simulink model "Simulation_6DOF"  (R2024a)
settings: Solver=ode4  StartTime=initial_time  StopTime=final_time  FixedStep=timestep  RelTol=1e-3
values from neighbouring files (symbols this model uses):
  aEarth = 0    [CodeTesting_6DOF.m]    (also in Constants_6DOF.m = 6378137; Constants_6DOFTesting.m = 6378137)
  alphaArray = [-30, -25, -20, -15, -10, -5, 0, 5, 10, 15, 20, 25, 30]    [CodeTesting_6DOF.m]    (also in Constants_6DOF.m; Constants_6DOFTesting.m)
  altitudeArray = [0, 1000, 2000, 3000, 4000, 5000, 6000, 7000, 8000, 9000, 10000, 15000, 20000,      25000, 30000, 35000, 40000, 45000, 50000, 55000, 60000]    [CodeTesting_6DOF.m]    (also in Constants_6DOF.m; Constants_6DOFTesting.m)
  AoA0Wind = 0    [CodeTesting_6DOF.m]    (also in Constants_6DOF.m = deg2rad(AoA0Wind); Constants_6DOFTesting.m = deg2rad(AoA0Wind))
  bEarth = 0    [CodeTesting_6DOF.m]    (also in Constants_6DOF.m = 6356752.3; Constants_6DOFTesting.m = 6356752.3)
  cD_3DArray = zeros(numAoAs, numMachs, numAltitudes)    [CodeTesting_6DOF.m]    (also in Constants_6DOF.m; Constants_6DOFTesting.m)
  cL_3DArray = zeros(numAoAs, numMachs, numAltitudes)    [CodeTesting_6DOF.m]    (also in Constants_6DOF.m; Constants_6DOFTesting.m)
  densityList = rhoList    [CodeTesting_6DOF.m]    (also in Constants_6DOF.m = usAtmosphere.x_; Constants_6DOFTesting.m = usAtmosphere.x_)
  heightsList = usAtmosphere.Z    [CodeTesting_6DOF.m]    (also in Constants_6DOF.m; Constants_6DOFTesting.m)
  Ixx = 10    [CodeTesting_6DOF.m]    (also in Constants_6DOF.m; Constants_6DOFTesting.m = 4.88094462)
  Ixz = 10    [CodeTesting_6DOF.m]    (also in Constants_6DOF.m = 1; Constants_6DOFTesting.m = 4.88094462)
  Iyy = 10    [CodeTesting_6DOF.m]    (also in Constants_6DOF.m; Constants_6DOFTesting.m = 4.88094462)
  Izz = 10    [CodeTesting_6DOF.m]    (also in Constants_6DOF.m; Constants_6DOFTesting.m = 4.88094462)
  latitude0 = pi/4    (= 0.785398163397)    [CodeTesting_6DOF.m]    (also in Constants_6DOF.m = deg2rad(latitude0); Constants_6DOFTesting.m = deg2rad(latitude0))
  longitude0 = pi/4    (= 0.785398163397)    [CodeTesting_6DOF.m]    (also in Constants_6DOF.m = deg2rad(longitude0); Constants_6DOFTesting.m = deg2rad(longitude0))
  m0 = 10    [CodeTesting_6DOF.m]    (also in Constants_6DOF.m = 50; Constants_6DOFTesting.m = 14.5939029)
  machArray = [0.5, 1.0, 1.5, 2.0, 2.5, 3.0, 3.5, 4.0, 4.5, 5.0, 5.5, 6.0, 6.5, 7.0, 7.5, 8.0,      8.5, 9.0, 9.5, 10.0]    [CodeTesting_6DOF.m]    (also in Constants_6DOF.m; Constants_6DOFTesting.m)
  omegaEarth = omega_earth    (= 7.2921159e-05)    [CodeTesting_6DOF.m]    (also in Constants_6DOF.m; Constants_6DOFTesting.m)
  p0Wind = 0    [CodeTesting_6DOF.m]    (also in Constants_6DOF.m = deg2rad(p0Wind))
  q0Wind = 0    [CodeTesting_6DOF.m]    (also in Constants_6DOF.m = deg2rad(q0Wind))
  r0Wind = 0    [CodeTesting_6DOF.m]    (also in Constants_6DOF.m = deg2rad(r0Wind))
  rEarth = r_earth    (= 6371008.8)    [CodeTesting_6DOF.m]    (also in Constants_6DOF.m; Constants_6DOFTesting.m)
  rollAngle0Wind = 0    [CodeTesting_6DOF.m]    (also in Constants_6DOF.m = deg2rad(rollAngle0Wind); Constants_6DOFTesting.m = deg2rad(rollAngle0Wind))
  sideslipAngle0Wind = 0    [CodeTesting_6DOF.m]    (also in Constants_6DOF.m = deg2rad(sideslipAngle0Wind); Constants_6DOFTesting.m = deg2rad(sideslipAngle0Wind))
  temperatureList = usAtmosphere.T    [CodeTesting_6DOF.m]    (also in Constants_6DOF.m; Constants_6DOFTesting.m)
  u0Wind = 5    [CodeTesting_6DOF.m]    (also in Constants_6DOF.m)
  v0Wind = 5    [CodeTesting_6DOF.m]    (also in Constants_6DOF.m = 0)
  w0Wind = 0    [CodeTesting_6DOF.m]    (also in Constants_6DOF.m)
  wingArea = 0    [CodeTesting_6DOF.m]    (also in Constants_6DOF.m = 50; Constants_6DOFTesting.m = 0.09290304)
  x0Wind = 5    [CodeTesting_6DOF.m]    (also in Constants_6DOF.m = 0)
  y0Wind = 5    [CodeTesting_6DOF.m]    (also in Constants_6DOF.m = 0)
  z0Wind = 5    [CodeTesting_6DOF.m]    (also in Constants_6DOF.m = 0)
settings Model: Creator=641893  LastModifiedBy=641893

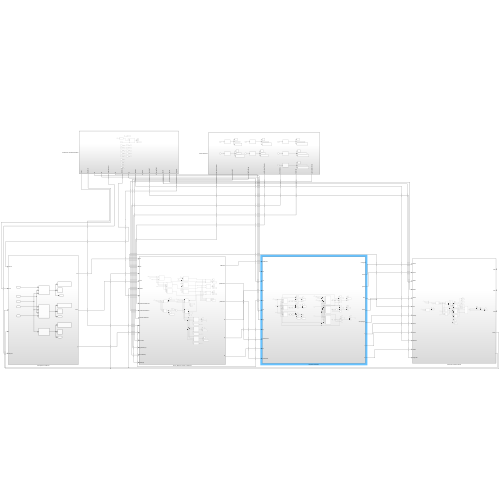
[thumbnail: Simulink's stored preview of the top-level diagram]
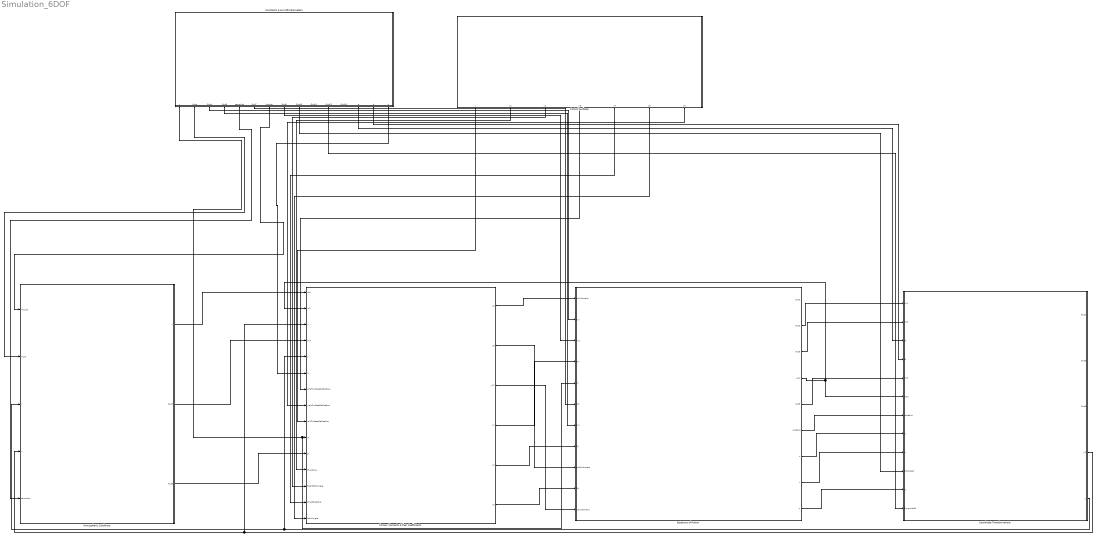
== system Simulation_6DOF ==
  Atmospheric Conditions : Subsystem
  Constants & Aircraft Parameters : Subsystem
  Control Surfaces : Subsystem
  Coordinate Transformations : Subsystem
  Equations of Motion : Subsystem
  "Forces, Moments & their Coefficients" : Subsystem
  wires:
  Atmospheric Conditions/1(y) -> "Forces, Moments & their Coefficients"/1(rho)
  Atmospheric Conditions/2(Out2) -> "Forces, Moments & their Coefficients"/4(In4)
  Atmospheric Conditions/3(Out3) -> "Forces, Moments & their Coefficients"/11(g)
  Equations of Motion/4(AoA) -> Coordinate Transformations/6(AoA), "Forces, Moments & their Coefficients"/2(In2)
  Constants & Aircraft Parameters/7(rhoList) -> Atmospheric Conditions/1(rhoList)
  Constants & Aircraft Parameters/2(hList) -> Atmospheric Conditions/2(hList)
  Constants & Aircraft Parameters/5(tempList) -> Atmospheric Conditions/5(tempList)
  Coordinate Transformations/4(y4) -> "Forces, Moments & their Coefficients"/3(v), Atmospheric Conditions/4(v)
  Coordinate Transformations/5(y) -> "Forces, Moments & their Coefficients"/5(y), Atmospheric Conditions/3(r)
  Constants & Aircraft Parameters/15(A) -> "Forces, Moments & their Coefficients"/6(A)
  Constants & Aircraft Parameters/1(y) -> Equations of Motion/5(m), "Forces, Moments & their Coefficients"/10(m)
  Control Surfaces/1(y) -> "Forces, Moments & their Coefficients"/9(rollSurfaceDeflection)
  Control Surfaces/4(y3) -> "Forces, Moments & their Coefficients"/7(pitchSurfaceDeflection)
  Control Surfaces/7(y6) -> "Forces, Moments & their Coefficients"/8(yawSurfaceDeflection)
  Control Surfaces/2(y1) -> "Forces, Moments & their Coefficients"/12(thrustAoA)
  Control Surfaces/3(y2) -> "Forces, Moments & their Coefficients"/13(flightPathAngle)
  Control Surfaces/5(y4) -> "Forces, Moments & their Coefficients"/14(thrustSideslip)
  Control Surfaces/6(y5) -> "Forces, Moments & their Coefficients"/15(bankAngle)
  "Forces, Moments & their Coefficients"/1(y5) -> Equations of Motion/1(rollMoment)
  "Forces, Moments & their Coefficients"/2(y8) -> Equations of Motion/9(pitchMoment)
  "Forces, Moments & their Coefficients"/3(y11) -> Equations of Motion/11(yawMoment)
  "Forces, Moments & their Coefficients"/6(y3) -> Equations of Motion/10(Fz)
  "Forces, Moments & their Coefficients"/5(y2) -> Equations of Motion/8(Fy)
  "Forces, Moments & their Coefficients"/4(y1) -> Equations of Motion/4(Fx)
  Constants & Aircraft Parameters/3(Out4) -> Equations of Motion/2(Ixx)
  Constants & Aircraft Parameters/4(Out5) -> Equations of Motion/7(Iyy)
  Constants & Aircraft Parameters/6(Out7) -> Equations of Motion/6(Izz)
  Constants & Aircraft Parameters/8(Out9) -> Equations of Motion/3(Ixz)
  Equations of Motion/2(Out2) -> Coordinate Transformations/1(In1)
  Equations of Motion/3(Out3) -> Coordinate Transformations/2(In3)
  Equations of Motion/5(Out5) -> Coordinate Transformations/5(In8)
  Equations of Motion/6(sideslip) -> Coordinate Transformations/7(sideslip)
  Equations of Motion/7(u) -> Coordinate Transformations/8(u)
  Equations of Motion/8(v) -> Coordinate Transformations/9(v)
  Equations of Motion/9(w) -> Coordinate Transformations/11(w)
  Constants & Aircraft Parameters/9(Out10) -> Coordinate Transformations/10(latitude0)
  Constants & Aircraft Parameters/13(a) -> Coordinate Transformations/3(a)
  Constants & Aircraft Parameters/14(b) -> Coordinate Transformations/4(b)
  Constants & Aircraft Parameters/11(Out12) -> Coordinate Transformations/12(longitude0)

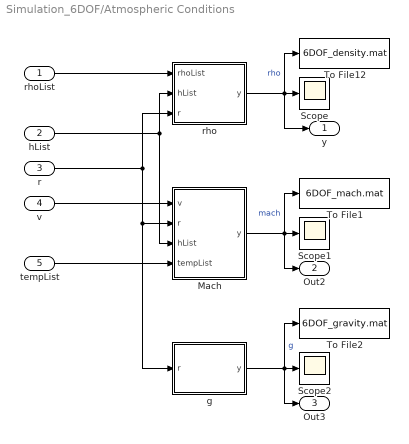
== system Simulation_6DOF/Atmospheric Conditions ==
  rhoList : Inport
  hList : Inport  Port=2
  r : Inport  Port=3
  v : Inport  Port=4
  tempList : Inport  Port=5
  Mach : MATLAB Function  TreatAsAtomicUnit=on
  Scope : Scope
  Scope1 : Scope
  Scope2 : Scope
  To File1 : ToFile  Filename=6DOF_mach.mat
  To File12 : ToFile  Filename=6DOF_density.mat
  To File2 : ToFile  Filename=6DOF_gravity.mat
  g : MATLAB Function  TreatAsAtomicUnit=on
  rho : MATLAB Function  TreatAsAtomicUnit=on
  y : Outport
  Out2 : Outport  Port=2
  Out3 : Outport  Port=3
  wires:
  rho/1(y) -> Scope/1, To File12/1, y/1  "rho"
  Mach/1(y) -> Scope1/1, To File1/1, Out2/1  "mach"
  g/1(y) -> To File2/1, Scope2/1, Out3/1  "g"
  hList/1 -> rho/2(hList), Mach/3(hList)
  v/1 -> Mach/1(v)
  tempList/1 -> Mach/4(tempList)
  r/1 -> rho/3(r), g/1(r), Mach/2(r)
  rhoList/1 -> rho/1(rhoList)

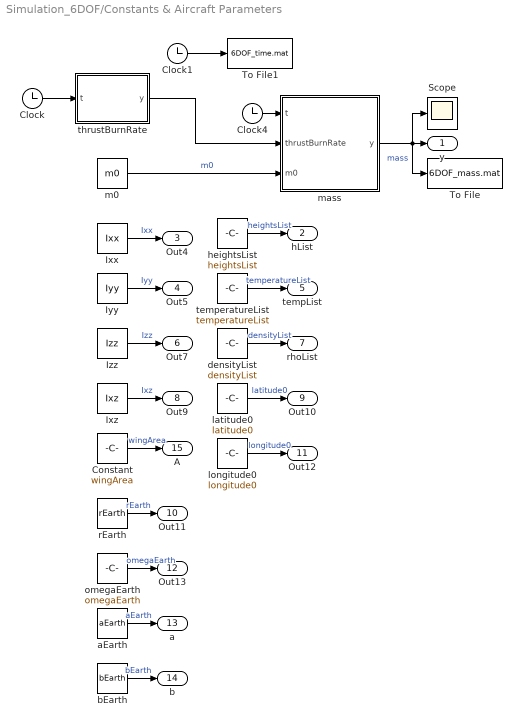
== system Simulation_6DOF/Constants & Aircraft Parameters ==
  Clock : Clock
  Clock1 : Clock
  Clock4 : Clock
  Constant : Constant  Value=wingArea
  Ixx : Constant  Value=Ixx
  Ixz : Constant  Value=Ixz
  Iyy : Constant  Value=Iyy
  Izz : Constant  Value=Izz
  Scope : Scope
  To File : ToFile  Filename=6DOF_mass.mat
  To File1 : ToFile  Filename=6DOF_time.mat
  aEarth : Constant  Value=aEarth
  bEarth : Constant  Value=bEarth
  densityList : Constant  Value=densityList
  heightsList : Constant  Value=heightsList
  latitude0 : Constant  Value=latitude0
  longitude0 : Constant  Value=longitude0
  m0 : Constant  Value=m0
  mass : MATLAB Function  TreatAsAtomicUnit=on
  omegaEarth : Constant  Value=omegaEarth
  rEarth : Constant  Value=rEarth
  temperatureList : Constant  Value=temperatureList
  thrustBurnRate : MATLAB Function  TreatAsAtomicUnit=on
  y : Outport
  hList : Outport  Port=2
  Out4 : Outport  Port=3
  Out5 : Outport  Port=4
  tempList : Outport  Port=5
  Out7 : Outport  Port=6
  rhoList : Outport  Port=7
  Out9 : Outport  Port=8
  Out10 : Outport  Port=9
  Out11 : Outport  Port=10
  Out12 : Outport  Port=11
  Out13 : Outport  Port=12
  a : Outport  Port=13
  b : Outport  Port=14
  A : Outport  Port=15
  wires:
  m0/1 -> mass/3(m0)  "m0"
  Clock4/1 -> mass/1(t)
  heightsList/1 -> hList/1  "heightsList"
  Clock/1 -> thrustBurnRate/1(t)
  omegaEarth/1 -> Out13/1  "omegaEarth"
  thrustBurnRate/1(y) -> mass/2(thrustBurnRate)
  rEarth/1 -> Out11/1  "rEarth"
  latitude0/1 -> Out10/1  "latitude0"
  mass/1(y) -> To File/1, Scope/1, y/1  "mass"
  aEarth/1 -> a/1  "aEarth"
  densityList/1 -> rhoList/1  "densityList"
  longitude0/1 -> Out12/1  "longitude0"
  bEarth/1 -> b/1  "bEarth"
  Izz/1 -> Out7/1  "Izz"
  Ixz/1 -> Out9/1  "Ixz"
  Ixx/1 -> Out4/1  "Ixx"
  temperatureList/1 -> tempList/1  "temperatureList"
  Iyy/1 -> Out5/1  "Iyy"
  Constant/1 -> A/1  "wingArea"
  Clock1/1 -> To File1/1

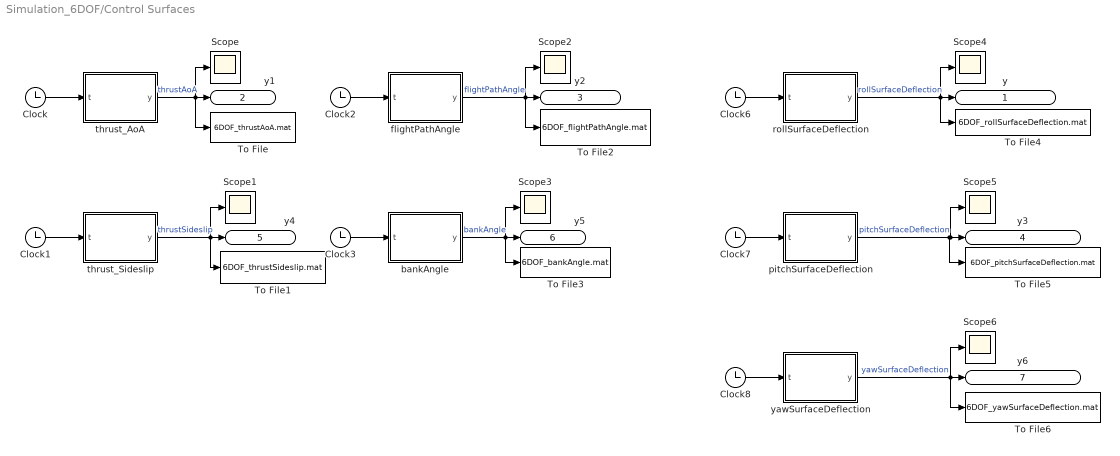
== system Simulation_6DOF/Control Surfaces ==
  Clock{,1..3,6..8} (7 alike) : Clock
  Scope{,1..6} (7 alike) : Scope
  To File : ToFile  Filename=6DOF_thrustAoA.mat
  To File1 : ToFile  Filename=6DOF_thrustSideslip.mat
  To File2 : ToFile  Filename=6DOF_flightPathAngle.mat
  To File3 : ToFile  Filename=6DOF_bankAngle.mat
  To File4 : ToFile  Filename=6DOF_rollSurfaceDeflection.mat
  To File5 : ToFile  Filename=6DOF_pitchSurfaceDeflection.mat
  To File6 : ToFile  Filename=6DOF_yawSurfaceDeflection.mat
  bankAngle : MATLAB Function  TreatAsAtomicUnit=on
  flightPathAngle : MATLAB Function  TreatAsAtomicUnit=on
  pitchSurfaceDeflection : MATLAB Function  TreatAsAtomicUnit=on
  rollSurfaceDeflection : MATLAB Function  TreatAsAtomicUnit=on
  thrust_AoA : MATLAB Function  TreatAsAtomicUnit=on
  thrust_Sideslip : MATLAB Function  TreatAsAtomicUnit=on
  yawSurfaceDeflection : MATLAB Function  TreatAsAtomicUnit=on
  y : Outport
  y1 : Outport  Port=2
  y2 : Outport  Port=3
  y3 : Outport  Port=4
  y4 : Outport  Port=5
  y5 : Outport  Port=6
  y6 : Outport  Port=7
  wires:
  Clock8/1 -> yawSurfaceDeflection/1(t)
  rollSurfaceDeflection/1(y) -> Scope4/1, y/1, To File4/1  "rollSurfaceDeflection"
  Clock1/1 -> thrust_Sideslip/1(t)
  bankAngle/1(y) -> Scope3/1, y5/1, To File3/1  "bankAngle"
  Clock6/1 -> rollSurfaceDeflection/1(t)
  Clock7/1 -> pitchSurfaceDeflection/1(t)
  pitchSurfaceDeflection/1(y) -> To File5/1, Scope5/1, y3/1  "pitchSurfaceDeflection"
  Clock2/1 -> flightPathAngle/1(t)
  thrust_AoA/1(y) -> Scope/1, y1/1, To File/1  "thrustAoA"
  Clock/1 -> thrust_AoA/1(t)
  Clock3/1 -> bankAngle/1(t)
  thrust_Sideslip/1(y) -> Scope1/1, y4/1, To File1/1  "thrustSideslip"
  flightPathAngle/1(y) -> Scope2/1, y2/1, To File2/1  "flightPathAngle"
  yawSurfaceDeflection/1(y) -> Scope6/1, y6/1, To File6/1  "yawSurfaceDeflection"

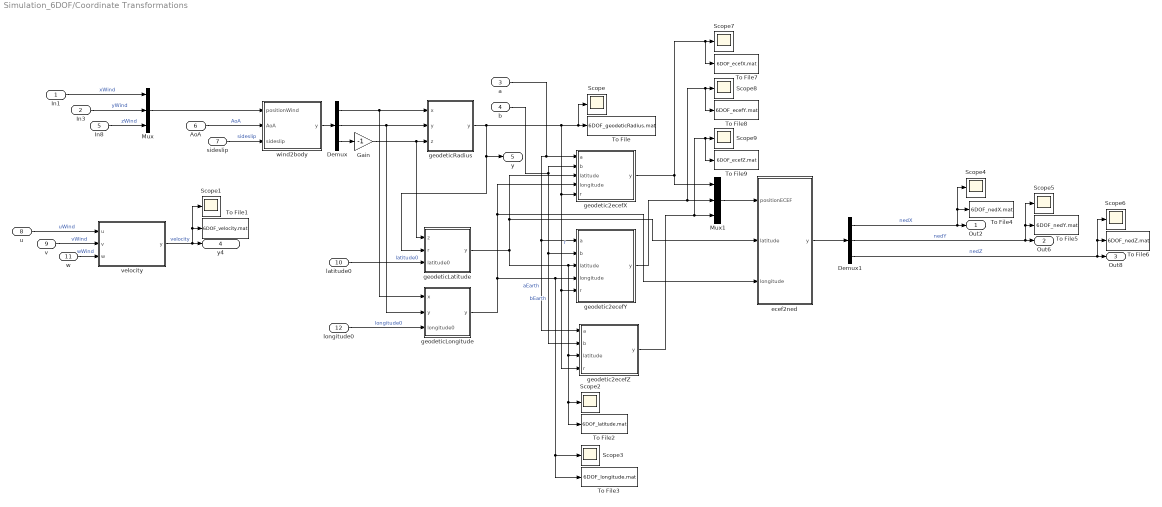
== system Simulation_6DOF/Coordinate Transformations ==
  In1 : Inport
  In3 : Inport  Port=2
  a : Inport  Port=3
  b : Inport  Port=4
  In8 : Inport  Port=5
  AoA : Inport  Port=6
  sideslip : Inport  Port=7
  u : Inport  Port=8
  v : Inport  Port=9
  latitude0 : Inport  Port=10
  w : Inport  Port=11
  longitude0 : Inport  Port=12
  Demux : Demux  Outputs=3
  Demux1 : Demux  Outputs=3
  Gain : Gain  Gain=-1
  Mux : Mux  Inputs=3
  Mux1 : Mux  Inputs=3
  Scope{,1..9} (10 alike) : Scope
  To File : ToFile  Filename=6DOF_geodeticRadius.mat
  To File1 : ToFile  Filename=6DOF_velocity.mat
  To File2 : ToFile  Filename=6DOF_latitude.mat
  To File3 : ToFile  Filename=6DOF_longitude.mat
  To File4 : ToFile  Filename=6DOF_nedX.mat
  To File5 : ToFile  Filename=6DOF_nedY.mat
  To File6 : ToFile  Filename=6DOF_nedZ.mat
  To File7 : ToFile  Filename=6DOF_ecefX.mat
  To File8 : ToFile  Filename=6DOF_ecefY.mat
  To File9 : ToFile  Filename=6DOF_ecefZ.mat
  ecef2ned : MATLAB Function  TreatAsAtomicUnit=on
  geodetic2ecefX : MATLAB Function  TreatAsAtomicUnit=on
  geodetic2ecefY : MATLAB Function  TreatAsAtomicUnit=on
  geodetic2ecefZ : MATLAB Function  TreatAsAtomicUnit=on
  geodeticLatitude : MATLAB Function  TreatAsAtomicUnit=on
  geodeticLongitude : MATLAB Function  TreatAsAtomicUnit=on
  geodeticRadius : MATLAB Function  TreatAsAtomicUnit=on
  velocity : MATLAB Function  TreatAsAtomicUnit=on
  wind2body : MATLAB Function  TreatAsAtomicUnit=on
  Out2 : Outport
  Out6 : Outport  Port=2
  Out8 : Outport  Port=3
  y4 : Outport  Port=4
  y : Outport  Port=5
  wires:
  Mux/1 -> wind2body/1(positionWind)
  geodeticRadius/1(y) -> y/1, geodeticLatitude/2(r), Scope/1, To File/1, geodetic2ecefX/5(r), geodetic2ecefY/5(r), geodetic2ecefZ/4(r)  "r"
  ecef2ned/1(y) -> Demux1/1
  v/1 -> velocity/2(v)  "vWind"
  u/1 -> velocity/1(u)  "uWind"
  sideslip/1 -> wind2body/3(sideslip)  "sideslip"
  Demux1/1 -> Scope4/1, To File4/1, Out2/1  "nedX"
  wind2body/1(y) -> Demux/1
  geodeticLongitude/1(y) -> geodetic2ecefY/4(longitude), Scope3/1, To File3/1, geodetic2ecefX/4(longitude), ecef2ned/3(longitude)
  b/1 -> geodetic2ecefX/2(b), geodetic2ecefY/2(b), geodetic2ecefZ/2(b)  "bEarth"
  longitude0/1 -> geodeticLongitude/3(longitude0)  "longitude0"
  Demux1/3 -> Scope6/1, To File6/1, Out8/1  "nedZ"
  Demux/3 -> Gain/1
  Demux1/2 -> Scope5/1, To File5/1, Out6/1  "nedY"
  latitude0/1 -> geodeticLatitude/3(latitude0)  "latitude0"
  a/1 -> geodetic2ecefX/1(a), geodetic2ecefZ/1(a), geodetic2ecefY/1(a)  "aEarth"
  w/1 -> velocity/3(w)  "wWind"
  AoA/1 -> wind2body/2(AoA)  "AoA"
  geodeticLatitude/1(y) -> geodetic2ecefZ/3(latitude), To File2/1, Scope2/1, geodetic2ecefY/3(latitude), geodetic2ecefX/3(latitude), ecef2ned/2(latitude)
  Demux/1 -> geodeticLongitude/1(x), geodeticRadius/1(x)
  Demux/2 -> geodeticRadius/2("y "), geodeticLongitude/2("y ")
  In8/1 -> Mux/3  "zWind"
  In1/1 -> Mux/1  "xWind"
  velocity/1(y) -> Scope1/1, To File1/1, y4/1  "velocity"
  In3/1 -> Mux/2  "yWind"
  Mux1/1 -> ecef2ned/1(positionECEF)
  geodetic2ecefX/1(y) -> To File7/1, Scope7/1, Mux1/1
  geodetic2ecefY/1(y) -> Mux1/2, To File8/1, Scope8/1
  geodetic2ecefZ/1(y) -> Mux1/3, To File9/1, Scope9/1
  Gain/1 -> geodeticLatitude/1(z), geodeticRadius/3(z)

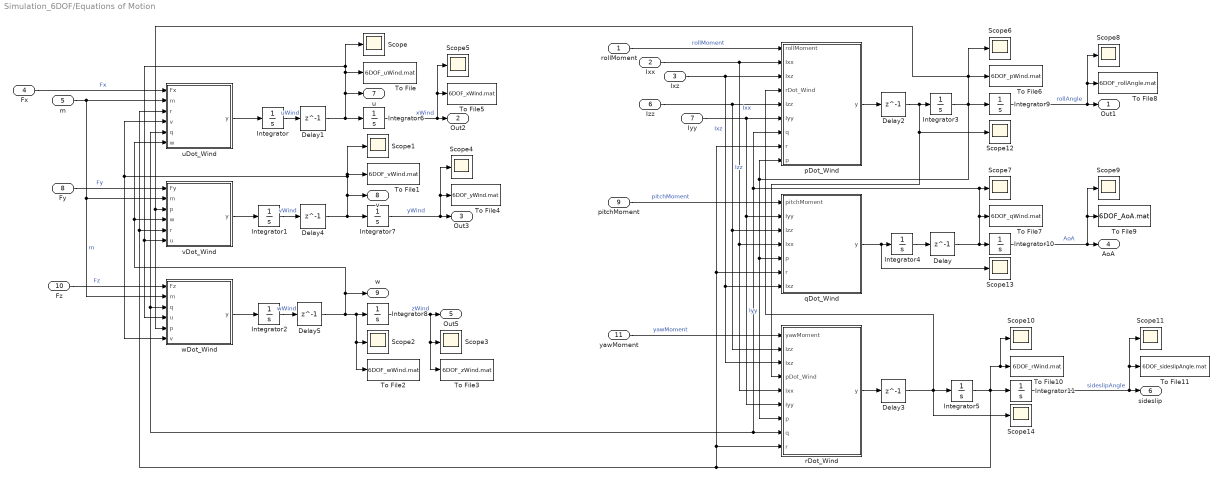
== system Simulation_6DOF/Equations of Motion ==
  rollMoment : Inport
  Ixx : Inport  Port=2
  Ixz : Inport  Port=3
  Fx : Inport  Port=4
  m : Inport  Port=5
  Izz : Inport  Port=6
  Iyy : Inport  Port=7
  Fy : Inport  Port=8
  pitchMoment : Inport  Port=9
  Fz : Inport  Port=10
  yawMoment : Inport  Port=11
  Delay{,1..5} (6 alike) : Delay  DelayLength=1  InitialCondition=0
  Integrator : Integrator  InitialCondition=u0Wind
  Integrator1 : Integrator  InitialCondition=v0Wind
  Integrator10 : Integrator  InitialCondition=AoA0Wind
  Integrator11 : Integrator  InitialCondition=sideslipAngle0Wind
  Integrator2 : Integrator  InitialCondition=w0Wind
  Integrator3 : Integrator  InitialCondition=p0Wind
  Integrator4 : Integrator  InitialCondition=q0Wind
  Integrator5 : Integrator  InitialCondition=r0Wind
  Integrator6 : Integrator  InitialCondition=x0Wind
  Integrator7 : Integrator  InitialCondition=y0Wind
  Integrator8 : Integrator  InitialCondition=z0Wind
  Integrator9 : Integrator  InitialCondition=rollAngle0Wind
  Scope{,1..14} (15 alike) : Scope
  To File : ToFile  Filename=6DOF_uWind.mat
  To File1 : ToFile  Filename=6DOF_vWind.mat
  To File10 : ToFile  Filename=6DOF_rWind.mat
  To File11 : ToFile  Filename=6DOF_sideslipAngle.mat
  To File2 : ToFile  Filename=6DOF_wWind.mat
  To File3 : ToFile  Filename=6DOF_zWind.mat
  To File4 : ToFile  Filename=6DOF_yWind.mat
  To File5 : ToFile  Filename=6DOF_xWind.mat
  To File6 : ToFile  Filename=6DOF_pWind.mat
  To File7 : ToFile  Filename=6DOF_qWind.mat
  To File8 : ToFile  Filename=6DOF_rollAngle.mat
  To File9 : ToFile  Filename=6DOF_AoA.mat
  pDot_Wind : MATLAB Function  TreatAsAtomicUnit=on
  qDot_Wind : MATLAB Function  TreatAsAtomicUnit=on
  rDot_Wind : MATLAB Function  TreatAsAtomicUnit=on
  uDot_Wind : MATLAB Function  TreatAsAtomicUnit=on
  vDot_Wind : MATLAB Function  TreatAsAtomicUnit=on
  wDot_Wind : MATLAB Function  TreatAsAtomicUnit=on
  Out1 : Outport
  Out2 : Outport  Port=2
  Out3 : Outport  Port=3
  AoA : Outport  Port=4
  Out5 : Outport  Port=5
  sideslip : Outport  Port=6
  u : Outport  Port=7
  v : Outport  Port=8
  w : Outport  Port=9
  wires:
  uDot_Wind/1(y) -> Integrator/1
  Fx/1 -> uDot_Wind/1(Fx)  "Fx"
  rollMoment/1 -> pDot_Wind/1(rollMoment)  "rollMoment"
  Integrator/1 -> Delay1/1  "uWind"
  Integrator2/1 -> Delay5/1  "wWind"
  Integrator1/1 -> Delay4/1  "vWind"
  Integrator11/1 -> Scope11/1, To File11/1, sideslip/1  "sideslipAngle"
  wDot_Wind/1(y) -> Integrator2/1
  Fy/1 -> vDot_Wind/1(Fy)  "Fy"
  vDot_Wind/1(y) -> Integrator1/1
  qDot_Wind/1(y) -> Scope13/1, Integrator4/1
  Ixx/1 -> pDot_Wind/2(Ixx), qDot_Wind/4(Ixx), rDot_Wind/5(Ixx)  "Ixx"
  Fz/1 -> wDot_Wind/1(Fz)  "Fz"
  Integrator7/1 -> Scope4/1, To File4/1, Out3/1  "yWind"
  Integrator10/1 -> Scope9/1, To File9/1, AoA/1  "AoA"
  pitchMoment/1 -> qDot_Wind/1(pitchMoment)  "pitchMoment"
  Integrator6/1 -> Scope5/1, To File5/1, Out2/1  "xWind"
  Integrator9/1 -> Scope8/1, To File8/1, Out1/1  "rollAngle"
  Izz/1 -> pDot_Wind/5(Izz), qDot_Wind/3(Izz), rDot_Wind/2(Izz)  "Izz"
  yawMoment/1 -> rDot_Wind/1(yawMoment)  "yawMoment"
  Iyy/1 -> pDot_Wind/6(Iyy), qDot_Wind/2(Iyy), rDot_Wind/6(Iyy)  "Iyy"
  Ixz/1 -> pDot_Wind/3(Ixz), qDot_Wind/7(Ixz), rDot_Wind/3(Ixz)  "Ixz"
  Integrator8/1 -> To File3/1, Scope3/1, Out5/1  "zWind"
  m/1 -> uDot_Wind/2(m), vDot_Wind/2(m), wDot_Wind/2(m)  "m"
  pDot_Wind/1(y) -> Delay2/1
  rDot_Wind/1(y) -> Delay3/1
  Integrator3/1 -> To File6/1, wDot_Wind/5(p), vDot_Wind/3(p), Scope6/1, qDot_Wind/5(p), rDot_Wind/7(p), pDot_Wind/9(p), Integrator9/1
  Integrator4/1 -> Delay/1
  Delay/1 -> rDot_Wind/8(q), wDot_Wind/3(q), uDot_Wind/5(q), pDot_Wind/7(q), Scope7/1, To File7/1, Integrator10/1
  Integrator5/1 -> Integrator11/1, Scope10/1, To File10/1, vDot_Wind/5(r), uDot_Wind/3(r), qDot_Wind/6(r), pDot_Wind/8(r), rDot_Wind/9(r)
  Delay1/1 -> vDot_Wind/6(u), wDot_Wind/4(u), Scope/1, To File/1, u/1, Integrator6/1
  Delay4/1 -> Integrator7/1, v/1, wDot_Wind/6(v), uDot_Wind/4(v), Scope1/1, To File1/1
  Delay5/1 -> w/1, vDot_Wind/4(w), uDot_Wind/6(w), To File2/1, Scope2/1, Integrator8/1
  Delay2/1 -> Scope12/1, rDot_Wind/4(pDot_Wind), Integrator3/1
  Delay3/1 -> pDot_Wind/4(rDot_Wind), Integrator5/1, Scope14/1

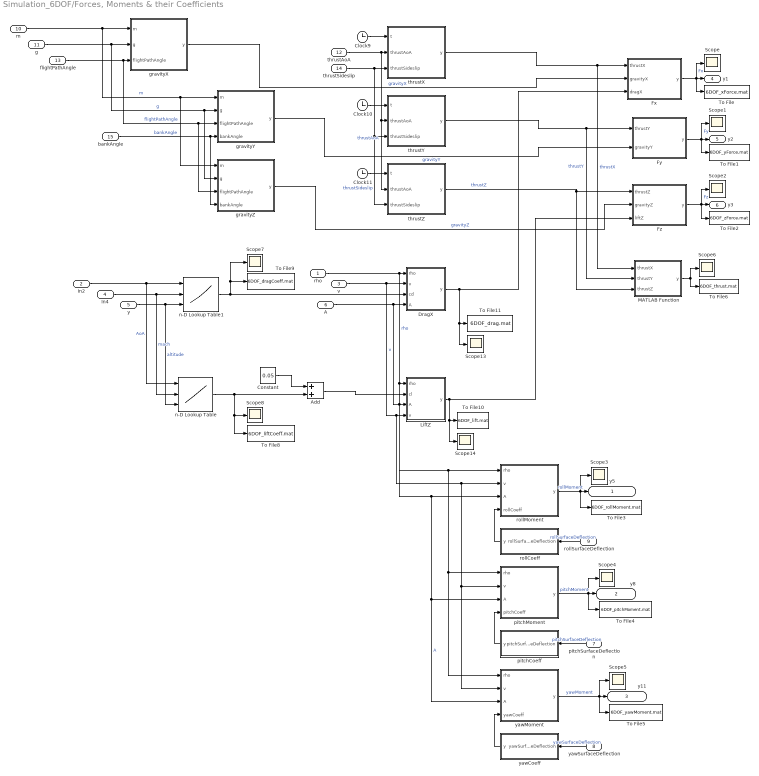
== system Simulation_6DOF/Forces, Moments & their Coefficients ==
  rho : Inport
  In2 : Inport  Port=2
  v : Inport  Port=3
  In4 : Inport  Port=4
  y : Inport  Port=5
  A : Inport  Port=6
  pitchSurfaceDeflection : Inport  Port=7
  yawSurfaceDeflection : Inport  Port=8
  rollSurfaceDeflection : Inport  Port=9
  m : Inport  Port=10
  g : Inport  Port=11
  thrustAoA : Inport  Port=12
  flightPathAngle : Inport  Port=13
  thrustSideslip : Inport  Port=14
  bankAngle : Inport  Port=15
  Add : Sum
  Clock10 : Clock
  Clock11 : Clock
  Clock9 : Clock
  Constant : Constant  Value=0.05
  DragX : MATLAB Function  TreatAsAtomicUnit=on
  Fx : MATLAB Function  TreatAsAtomicUnit=on
  Fy : MATLAB Function  TreatAsAtomicUnit=on
  Fz : MATLAB Function  TreatAsAtomicUnit=on
  LiftZ : MATLAB Function  TreatAsAtomicUnit=on
  MATLAB Function : MATLAB Function  TreatAsAtomicUnit=on
  Scope{,1..8,13..14} (11 alike) : Scope
  To File : ToFile  Filename=6DOF_xForce.mat
  To File1 : ToFile  Filename=6DOF_yForce.mat
  To File10 : ToFile  Filename=6DOF_lift.mat
  To File11 : ToFile  Filename=6DOF_drag.mat
  To File2 : ToFile  Filename=6DOF_zForce.mat
  To File3 : ToFile  Filename=6DOF_rollMoment.mat
  To File4 : ToFile  Filename=6DOF_pitchMoment.mat
  To File5 : ToFile  Filename=6DOF_yawMoment.mat
  To File6 : ToFile  Filename=6DOF_thrust.mat
  To File8 : ToFile  Filename=6DOF_liftCoeff.mat
  To File9 : ToFile  Filename=6DOF_dragCoeff.mat
  gravityX : MATLAB Function  TreatAsAtomicUnit=on
  gravityY : MATLAB Function  TreatAsAtomicUnit=on
  gravityZ : MATLAB Function  TreatAsAtomicUnit=on
  n-D Lookup Table : Lookup_n-D  NumberOfTableDimensions=3  BreakpointsForDimension1=alphaArray  BreakpointsForDimension2=machArray  BreakpointsForDimension3=altitudeArray  IndexSearchMethod=Linear search  Table=cL_3DArray  InterpMethod=Linear Lagrange  InternalRulePriority=Speed  RndMeth=Simplest
      settings: InputPortMap=u0,u1,u2
  n-D Lookup Table1 : Lookup_n-D  NumberOfTableDimensions=3  BreakpointsForDimension1=alphaArray  BreakpointsForDimension2=machArray  BreakpointsForDimension3=altitudeArray  IndexSearchMethod=Linear search  Table=cD_3DArray  InterpMethod=Linear Lagrange  InternalRulePriority=Speed  RndMeth=Simplest
      settings: InputPortMap=u0,u1,u2
  pitchCoeff : MATLAB Function  TreatAsAtomicUnit=on
  pitchMoment : MATLAB Function  TreatAsAtomicUnit=on
  rollCoeff : MATLAB Function  TreatAsAtomicUnit=on
  rollMoment : MATLAB Function  TreatAsAtomicUnit=on
  thrustX : MATLAB Function  TreatAsAtomicUnit=on
  thrustY : MATLAB Function  TreatAsAtomicUnit=on
  thrustZ : MATLAB Function  TreatAsAtomicUnit=on
  yawCoeff : MATLAB Function  TreatAsAtomicUnit=on
  yawMoment : MATLAB Function  TreatAsAtomicUnit=on
  y5 : Outport
  y8 : Outport  Port=2
  y11 : Outport  Port=3
  y1 : Outport  Port=4
  y2 : Outport  Port=5
  y3 : Outport  Port=6
  wires:
  Clock11/1 -> thrustZ/1(t)
  n-D Lookup Table/1 -> Add/2, To File8/1, Scope8/1
  LiftZ/1(y) -> Fz/3(liftZ), Scope14/1, To File10/1
  n-D Lookup Table1/1 -> Scope7/1, To File9/1, DragX/3(cd)
  v/1 -> DragX/2(v), LiftZ/4(v), rollMoment/2(v), yawMoment/2(v), pitchMoment/2(v)  "v"
  DragX/1(y) -> Fx/3(dragX), Scope13/1, To File11/1
  y/1 -> n-D Lookup Table1/3, n-D Lookup Table/3  "altitude"
  rollMoment/1(y) -> Scope3/1, y5/1, To File3/1  "rollMoment"
  g/1 -> gravityX/2(g), gravityY/2(g), gravityZ/2(g)  "g"
  yawSurfaceDeflection/1 -> yawCoeff/1(yawSurfaceDeflection)  "yawSurfaceDeflection"
  yawMoment/1(y) -> To File5/1, Scope5/1, y11/1  "yawMoment"
  Clock9/1 -> thrustX/1(t)
  rho/1 -> rollMoment/1(rho), yawMoment/1(rho), pitchMoment/1(rho), LiftZ/1(rho), DragX/1(rho)  "rho"
  Clock10/1 -> thrustY/1(t)
  rollSurfaceDeflection/1 -> rollCoeff/1(rollSurfaceDeflection)  "rollSurfaceDeflection"
  m/1 -> gravityX/1(m), gravityY/1(m), gravityZ/1(m)  "m"
  In2/1 -> n-D Lookup Table1/1, n-D Lookup Table/1  "AoA"
  A/1 -> DragX/4(A), rollMoment/3(A), yawMoment/3(A), pitchMoment/3(A), LiftZ/3(A)  "A"
  thrustAoA/1 -> thrustZ/2(thrustAoA), thrustY/2(thrustAoA), thrustX/2(thrustAoA)  "thrustAoA"
  bankAngle/1 -> gravityZ/4(bankAngle), gravityY/4(bankAngle)  "bankAngle"
  flightPathAngle/1 -> gravityZ/3(flightPathAngle), gravityY/3(flightPathAngle), gravityX/3(flightPathAngle)  "flightPathAngle"
  In4/1 -> n-D Lookup Table1/2, n-D Lookup Table/2  "mach"
  thrustSideslip/1 -> thrustX/3(thrustSideslip), thrustY/3(thrustSideslip), thrustZ/3(thrustSideslip)  "thrustSideslip"
  pitchMoment/1(y) -> Scope4/1, y8/1, To File4/1  "pitchMoment"
  pitchSurfaceDeflection/1 -> pitchCoeff/1(pitchSurfaceDeflection)  "pitchSurfaceDeflection"
  pitchCoeff/1(y) -> pitchMoment/4(pitchCoeff)
  rollCoeff/1(y) -> rollMoment/4(rollCoeff)
  yawCoeff/1(y) -> yawMoment/4(yawCoeff)
  Fx/1(y) -> Scope/1, y1/1, To File/1  "Fx"
  thrustX/1(y) -> MATLAB Function/1(thrustX), Fx/1(thrustX)  "thrustX"
  gravityX/1(y) -> Fx/2(gravityX)  "gravityX"
  thrustY/1(y) -> Fy/1(thrustY), MATLAB Function/2(thrustY)  "thrustY"
  gravityY/1(y) -> Fy/2(gravityY)  "gravityY"
  Fy/1(y) -> Scope1/1, y2/1, To File1/1  "Fy"
  Fz/1(y) -> Scope2/1, y3/1, To File2/1  "Fz"
  thrustZ/1(y) -> Fz/1(thrustZ), MATLAB Function/3(thrustZ)  "thrustZ"
  gravityZ/1(y) -> Fz/2(gravityZ)  "gravityZ"
  MATLAB Function/1(y) -> To File6/1, Scope6/1
  Add/1 -> LiftZ/2(cl)
  Constant/1 -> Add/1

== matlab function Simulation_6DOF/Control Surfaces/pitchSurfaceDeflection ==
  data: t input; y output
function y = fcn(t)

pitchSurfaceDeflection = 0.0;

if t > 5 && t < 15
    pitchSurfaceDeflection = 0.001;
end

if t > 20 && t < 25
    pitchSurfaceDeflection = -0.001;
end


y = pitchSurfaceDeflection;

== matlab function Simulation_6DOF/Control Surfaces/yawSurfaceDeflection ==
  data: t input; y output
function y = fcn(t)

yawSurfaceDeflection = 0;

y = yawSurfaceDeflection;

== matlab function Simulation_6DOF/Forces, Moments & their Coefficients/thrustX ==
  data: t input; y output; thrustAoA input; thrustSideslip input
function y = fcn(t, thrustAoA, thrustSideslip)

thrust = 0;

thrust = thrust * cos(thrustAoA) * cos(thrustSideslip);

y = thrust;

== matlab function Simulation_6DOF/Atmospheric Conditions/Mach ==
  data: v input; y output; r input; hList input; tempList input
function y = fcn(v, r, hList, tempList)

gamma = 1.4;
rGas = 287.05;

r = r / 10^3;

if r >= 0
    temp = interp1(hList, tempList, r);
    a = sqrt(gamma * rGas * temp);
    y = v/a;
else
    temp = 0;
    y = 0;
end

== matlab function Simulation_6DOF/Forces, Moments & their Coefficients/thrustY ==
  data: t input; y output; thrustAoA input; thrustSideslip input
function y = fcn(t, thrustAoA, thrustSideslip)

thrust = 0;

thrust = thrust * cos(thrustAoA) * sin(thrustSideslip);

y = thrust;

== matlab function Simulation_6DOF/Forces, Moments & their Coefficients/thrustZ ==
  data: t input; y output; thrustAoA input; thrustSideslip input
function y = fcn(t, thrustAoA, thrustSideslip)

thrust = 0;

thrust = -1 * thrust * sin(thrustAoA);

y = thrust;

== matlab function Simulation_6DOF/Forces, Moments & their Coefficients/gravityX ==
  data: m input; y output; g input; flightPathAngle input
function y = fcn(m, g, flightPathAngle)

gravity = -1 * m * g * sin(flightPathAngle);

y = gravity;

== matlab function Simulation_6DOF/Control Surfaces/thrust_Sideslip ==
  data: t input; y output
function y = fcn(t)

thrustSideslip = 0;

y = thrustSideslip;

== matlab function Simulation_6DOF/Forces, Moments & their Coefficients/gravityY ==
  data: m input; y output; g input; flightPathAngle input; bankAngle input
function y = fcn(m, g, flightPathAngle, bankAngle)

gravity = m * g * cos(flightPathAngle) * sin(bankAngle);

y = gravity;

== matlab function Simulation_6DOF/Forces, Moments & their Coefficients/gravityZ ==
  data: m input; y output; g input; flightPathAngle input; bankAngle input
function y = fcn(m, g, flightPathAngle, bankAngle)

gravity = m * g * cos(flightPathAngle) * cos(bankAngle);

y = gravity;

== matlab function Simulation_6DOF/Forces, Moments & their Coefficients/rollMoment ==
  data: rho input; y output; v input; A input; rollCoeff input
function y = fcn(rho, v, A, rollCoeff)

rollMoment = 0.5 * rho * v^2 * A * rollCoeff;

y = rollMoment;

== matlab function Simulation_6DOF/Forces, Moments & their Coefficients/pitchMoment ==
  data: rho input; y output; v input; A input; pitchCoeff input
function y = fcn(rho, v, A, pitchCoeff)

pitchMoment = 0.5 * rho * v^2 * A * pitchCoeff;

y = pitchMoment;

== matlab function Simulation_6DOF/Forces, Moments & their Coefficients/yawMoment ==
  data: rho input; y output; v input; A input; yawCoeff input
function y = fcn(rho, v, A, yawCoeff)

yawMoment = 0.5 * rho * v^2 * A * yawCoeff;

y = yawMoment;

== matlab function Simulation_6DOF/Equations of Motion/uDot_Wind ==
  data: Fx input; y output; m input; r input; v input; q input; w input
function y = fcn(Fx, m, r, v, q, w)

uDot_Wind = (Fx/m) + r * v - q * w;

y = uDot_Wind;

== matlab function Simulation_6DOF/Equations of Motion/vDot_Wind ==
  data: Fy input; y output; m input; p input; w input; r input; u input
function y = fcn(Fy, m, p, w, r,  u)

vDot_Wind = (Fy / m) + p * w - r * u;

y = vDot_Wind;

== matlab function Simulation_6DOF/Control Surfaces/thrust_AoA ==
  data: t input; y output
function y = fcn(t)

thrustAoA = 0;

y = thrustAoA;

== matlab function Simulation_6DOF/Equations of Motion/wDot_Wind ==
  data: Fz input; y output; m input; q input; u input; p input; v input
function y = fcn(Fz, m, q, u, p, v)

vDot_Wind = (Fz / m) + q * u - p * v;

y = vDot_Wind;

== matlab function Simulation_6DOF/Equations of Motion/pDot_Wind ==
  data: rollMoment input; y output; Ixx input; Ixz input; rDot_Wind input; Izz input; Iyy input; q input; r input; p input
function y = fcn(rollMoment, Ixx, Ixz, rDot_Wind, Izz, Iyy, q, r, p)

pDot_Wind = (1/Ixx) * (Ixz * rDot_Wind - (Izz - Iyy) * q * r + Ixz * p * q - rollMoment);

y = pDot_Wind;

== matlab function Simulation_6DOF/Equations of Motion/qDot_Wind ==
  data: pitchMoment input; Iyy input; Izz input; y output; Ixx input; p input; r input; Ixz input
function y = fcn(pitchMoment, Iyy, Izz, Ixx, p, r, Ixz)

pDot_Wind = (1/Iyy) * ( (Izz - Ixx) * p * r + Ixz * (p^2 - r^2) - pitchMoment);

y = pDot_Wind;

== matlab function Simulation_6DOF/Equations of Motion/rDot_Wind ==
  data: yawMoment input; Izz input; Ixz input; pDot_Wind input; y output; Ixx input; Iyy input; p input; q input; r input
function y = fcn(yawMoment, Izz, Ixz, pDot_Wind, Ixx, Iyy, p, q, r)

rDot_Wind = (1/Izz) * (Ixz * pDot_Wind - (Ixx - Iyy) * p * q + Ixz * q * r - yawMoment);

y = rDot_Wind;

== matlab function Simulation_6DOF/Constants & Aircraft Parameters/mass ==
  data: t input; y output; thrustBurnRate input; m0 input
function y = fcn(t, thrustBurnRate, m0)

mass = m0 - thrustBurnRate * t;

y = mass;

== matlab function Simulation_6DOF/Control Surfaces/flightPathAngle ==
  data: t input; y output
function y = fcn(t)

flightPathAngle = 0;

y = flightPathAngle;

== matlab function Simulation_6DOF/Coordinate Transformations/geodeticRadius ==
  data: x input; y output; y input; z input
function y = fcn(x, y, z)

radiusGeodetic = sqrt(x^2 + y^2 + z^2);

y = radiusGeodetic;

== matlab function Simulation_6DOF/Coordinate Transformations/geodeticLatitude ==
  data: z input; y output; r input; latitude0 input
function y = fcn(z, r, latitude0)

latitude = asin(z/r) + latitude0;

y = latitude;

== matlab function Simulation_6DOF/Coordinate Transformations/geodeticLongitude ==
  data: x input; y output; y input; longitude0 input
function y = fcn(x, y, longitude0)

longitude = atan2(y,x) + longitude0;

y = longitude;

== matlab function Simulation_6DOF/Coordinate Transformations/geodetic2ecefX ==
  data: a input; y output; b input; latitude input; longitude input; r input
function y = fcn(a, b, latitude, longitude, r)

e = sqrt(1 - b^2/a^2);
nPhi = a * (1 - e^2 * (sin(latitude))^2);

ecefX = (nPhi + r) * cos(latitude) * cos(longitude);

y = ecefX;

== matlab function Simulation_6DOF/Coordinate Transformations/geodetic2ecefY ==
  data: a input; y output; b input; latitude input; longitude input; r input
function y = fcn(a, b, latitude, longitude, r)

e = sqrt(1 - b^2/a^2);
nPhi = a * (1 - e^2 * (sin(latitude))^2);

ecefY = (nPhi + r) * cos(latitude) * sin(longitude);

y = ecefY;

== matlab function Simulation_6DOF/Coordinate Transformations/geodetic2ecefZ ==
  data: a input; y output; b input; latitude input; r input
function y = fcn(a, b, latitude, r)

e = sqrt(1 - b^2/a^2);
nPhi = a * (1 - e^2 * (sin(latitude))^2);

ecefZ = ((1 - e^2) * nPhi + r) * sin(latitude);

y = ecefZ;

== matlab function Simulation_6DOF/Coordinate Transformations/ecef2ned ==
  data: positionECEF input; y output; latitude input; longitude input
function y = fcn(positionECEF, latitude, longitude)

rotationMatrix = [-sin(latitude) * cos(longitude) -sin(latitude) * sin(longitude) cos(latitude); -sin(longitude) cos(longitude) 0; -cos(latitude) * cos(longitude) -cos(latitude) * sin(longitude) sin(latitude)];

nedPosition = rotationMatrix * positionECEF;

y = nedPosition;

== matlab function Simulation_6DOF/Control Surfaces/bankAngle ==
  data: t input; y output
function y = fcn(t)

bankAngle = 0;

y = bankAngle;

== matlab function Simulation_6DOF/Forces, Moments & their Coefficients/rollCoeff ==
  data: rollSurfaceDeflection input; y output
function y = fcn(rollSurfaceDeflection)

rollCoeff = rollSurfaceDeflection;

y = rollCoeff;

== matlab function Simulation_6DOF/Forces, Moments & their Coefficients/pitchCoeff ==
  data: pitchSurfaceDeflection input; y output
function y = fcn(pitchSurfaceDeflection)

pitchCoeff = pitchSurfaceDeflection;

y = pitchCoeff;

== matlab function Simulation_6DOF/Forces, Moments & their Coefficients/yawCoeff ==
  data: yawSurfaceDeflection input; y output
function y = fcn(yawSurfaceDeflection)

yawCoeff = yawSurfaceDeflection;

y = yawCoeff;

== matlab function Simulation_6DOF/Constants & Aircraft Parameters/thrustBurnRate ==
  data: t input; y output
function y = fcn(t)

thrustBurnRate = 0;

y = thrustBurnRate;

== matlab function Simulation_6DOF/Forces, Moments & their Coefficients/Fx ==
  data: thrustX input; y output; gravityX input; dragX input
function y = fcn(thrustX, gravityX, dragX)

thrustX = dragX;
xForce = thrustX + gravityX - dragX;

y = xForce;

== matlab function Simulation_6DOF/Forces, Moments & their Coefficients/Fy ==
  data: thrustY input; y output; gravityY input
function y = fcn(thrustY, gravityY)

yForce = thrustY + gravityY;

y = yForce;

== matlab function Simulation_6DOF/Forces, Moments & their Coefficients/Fz ==
  data: thrustZ input; y output; gravityZ input; liftZ input
function y = fcn(thrustZ, gravityZ, liftZ)

liftZ = gravityZ;
zForce = thrustZ + gravityZ - liftZ;

y = zForce;

== matlab function Simulation_6DOF/Forces, Moments & their Coefficients/MATLAB Function ==
  data: thrustX input; y output; thrustY input; thrustZ input
function y = fcn(thrustX, thrustY, thrustZ)

thrustMagnitude = sqrt(thrustX^2 + thrustY^2 + thrustZ^2);

y = thrustMagnitude;

== matlab function Simulation_6DOF/Coordinate Transformations/velocity ==
  data: u input; y output; v input; w input
function y = fcn(u, v, w)

velocity = sqrt(u^2 + v^2 + w^2);

y = velocity;

== matlab function Simulation_6DOF/Coordinate Transformations/wind2body ==
  data: positionWind input; y output; AoA input; sideslip input
function y = fcn(positionWind, AoA, sideslip)

rotationMatrix = [cos(AoA) * cos(sideslip) -cos(AoA) * sin(sideslip) -sin(AoA); sin(sideslip) cos(sideslip) 0; sin(AoA) * cos(sideslip) -sin(AoA) * sin(sideslip) cos(AoA)];

positionBody = rotationMatrix * positionWind;

y = positionBody;

== matlab function Simulation_6DOF/Control Surfaces/rollSurfaceDeflection ==
  data: t input; y output
function y = fcn(t)

rollSurfaceDeflection = 0.0;

y = rollSurfaceDeflection;

== matlab function Simulation_6DOF/Forces, Moments & their Coefficients/LiftZ ==
  data: rho input; y output; cl input; A input; v input
function y = fcn(rho, cl, A, v)

y = 0.5 * rho * v^2 * A * cl;

== matlab function Simulation_6DOF/Forces, Moments & their Coefficients/DragX ==
  data: rho input; y output; v input; cd input; A input
function y = fcn(rho, v, cd, A)

Drag = 0.5 * rho * v^2 * A * cd;

y = Drag;

== matlab function Simulation_6DOF/Atmospheric Conditions/g ==
  data: y output; r input
function y = fcn(r)

mu_earth = 3.96272 * 10^14;
rE = 6378140;

y = mu_earth / (rE + r)^2;

== matlab function Simulation_6DOF/Atmospheric Conditions/rho ==
  data: rhoList input; hList input; r input; y output
function y = fcn(rhoList, hList, r)

r = r / 10^3;

if r >= 0
    density = interp1(hList, rhoList, r);
else
    density = 0;
end


y = density;
